simulink model "tut2"  (R2025b)
settings: Solver=VariableStepAuto  StartTime=0.0  StopTime=100.0  RelTol=1e-3
libraries: commrflib2 x1
settings Model: Creator=anish  LastModifiedBy=anish

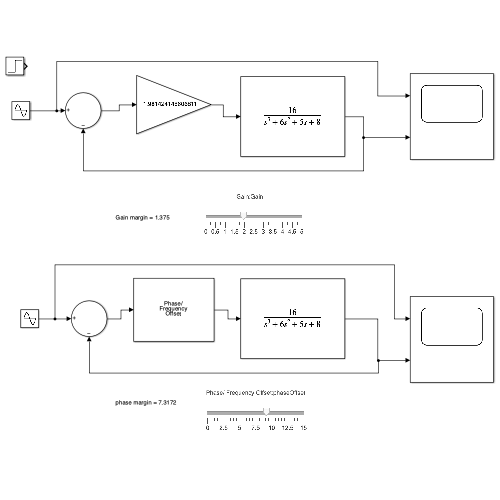
[thumbnail: Simulink's stored preview of the top-level diagram]
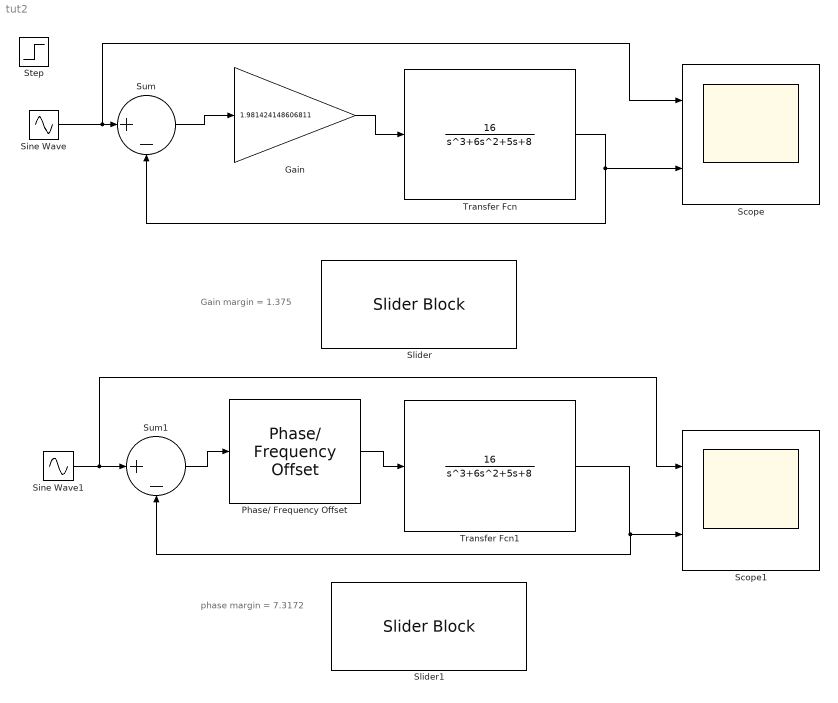
== system tut2 ==
  note: phase margin = 7.3172
  note: Gain margin = 1.375
  Gain : Gain  Gain=1.981424148606811
  Phase/ Frequency Offset : commrflib2/Phase// Frequency Offset  phaseOffset=9.195046439628483  freqPort=off  freqOffset=0
  Scope : Scope  NumInputPorts=2
      settings: ActiveDisplayYMinimum=-37.000208874145706  ActiveDisplayYMaximum=26.631615792010138
  Scope1 : Scope  NumInputPorts=2
      settings: ActiveDisplayYMinimum=-37.000208874145706  ActiveDisplayYMaximum=26.631615792010138
  Sine Wave : Sin  SampleTime=0
  Sine Wave1 : Sin  SampleTime=0
  Slider : SliderBlock  ScaleMax=5
  Slider1 : SliderBlock  ScaleMax=15
  Step : Step  SampleTime=0
  Sum : Sum  Inputs=|+-
  Sum1 : Sum  Inputs=|+-
  Transfer Fcn : TransferFcn  Numerator=[16]  Denominator=[1 6 5 8]
  Transfer Fcn1 : TransferFcn  Numerator=[16]  Denominator=[1 6 5 8]
  wires:
  Gain/1 -> Transfer Fcn/1
  Sum/1 -> Gain/1
  Transfer Fcn/1 -> Scope/2, Sum/2
  Sine Wave/1 -> Scope/1, Sum/1
  Sum1/1 -> Phase/ Frequency Offset/1
  Sine Wave1/1 -> Scope1/1, Sum1/1
  Transfer Fcn1/1 -> Sum1/2, Scope1/2
  Phase/ Frequency Offset/1 -> Transfer Fcn1/1
